simulink model "gnc_1__1_1"  (R2025b)
settings: Solver=VariableStepAuto  StartTime=0.0  StopTime=10.0  RelTol=1e-3
libraries: simulink_extras x4
settings Model: Creator=hp  LastModifiedBy=ADMIN

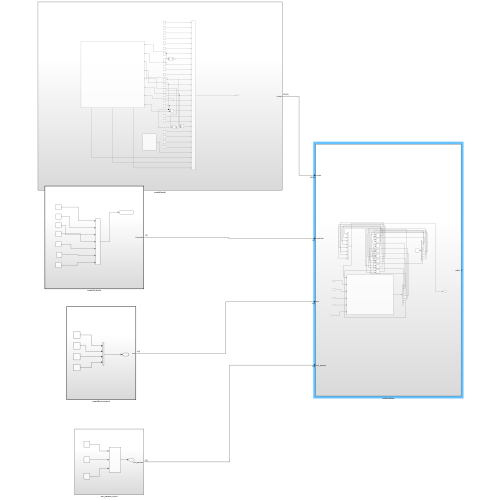
[thumbnail: Simulink's stored preview of the top-level diagram]
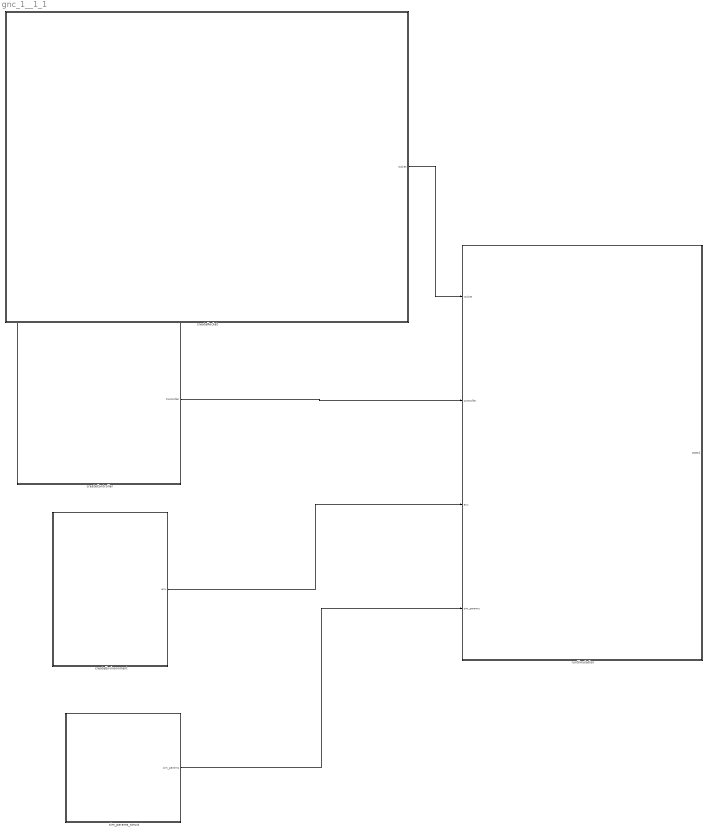
== system gnc_1__1_1 ==
  createController : Subsystem  TreatAsAtomicUnit=on
  createEnvironnment : Subsystem  TreatAsAtomicUnit=on
  createRocket : Subsystem
  runSimulation : Subsystem
  sim_params_struct : Subsystem
  wires:
  sim_params_struct/1(sim_params) -> runSimulation/4(sim_params)
  createEnvironnment/1(env) -> runSimulation/3(env)
  createController/1(Controller) -> runSimulation/2(controller)
  createRocket/1(rocket) -> runSimulation/1(rocket)

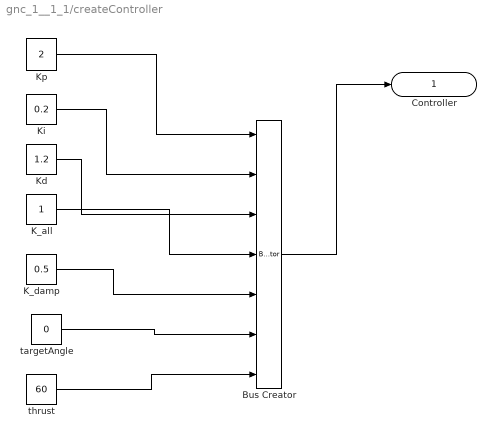
== system gnc_1__1_1/createController ==
  Bus Creator : BusCreator  Inputs=7
  K_all : Constant
  K_damp : Constant  Value=0.5
  Kd : Constant  Value=1.2
  Ki : Constant  Value=0.2
  Kp : Constant  Value=2
  targetAngle : Constant  Value=0
  thrust : Constant  Value=60
  Controller : Outport
  wires:
  Kp/1 -> Bus Creator/1
  Ki/1 -> Bus Creator/2
  Kd/1 -> Bus Creator/3
  K_all/1 -> Bus Creator/4
  K_damp/1 -> Bus Creator/5
  targetAngle/1 -> Bus Creator/6
  thrust/1 -> Bus Creator/7
  Bus Creator/1 -> Controller/1

== system gnc_1__1_1/createEnvironnment ==
  Bus Creator : BusCreator  Inputs=4
  P0 : Constant  Value=101325
  RHO0 : Constant  Value=1.225
  T0 : Constant  Value=288.15
  g : Constant  Value=9.81
  env : Outport
  wires:
  Bus Creator/1 -> env/1
  g/1 -> Bus Creator/1
  T0/1 -> Bus Creator/2
  P0/1 -> Bus Creator/3
  RHO0/1 -> Bus Creator/4

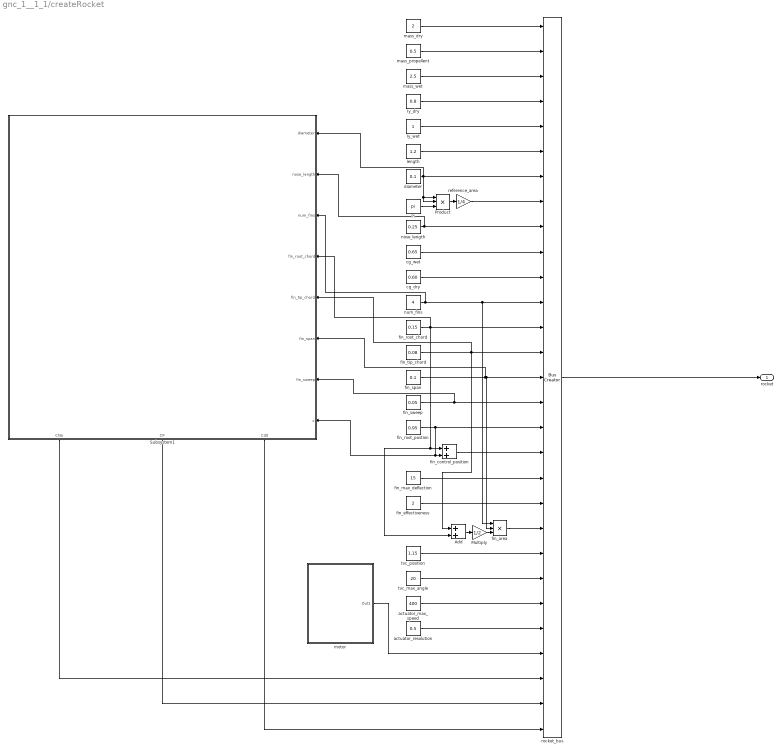
== system gnc_1__1_1/createRocket ==
  Add : Sum
  Iy_dry : Constant  Value=0.8
  Iy_wet : Constant
  Multiply : Gain  Gain=1/2
  Pi : Constant  Value=pi  OutDataTypeStr=Inherit: Inherit via back propagation
  Product : Product  Inputs=3
  Subsystem1 : Subsystem
      settings: PortSchema="{\"entries\":[{\"content\":{\"sides\":[{\"content\":{},\"type\":\"ConnectorPlacement.EquallySpacedRectSide\",\"uuid\":\"6679e0f2-b643-4e75-9411-8b79dd5cee92\"},{\"content\":{\"connectorIds\":[\"In1\",\"In2\",\"In3\",\"In4\",\"In5\",\"In6\",\"In7\",\"In8\"],\"side\":\"RIGHT\"},\"type\":\"ConnectorPlacement.EquallySpacedRectSide\",\"uuid\":\"6d3ac53c-a821-4766-a15e-70655263746a\"},{\"content\":{\"side\":\"TOP\"},\"type\":\"ConnectorPlacement.EquallySpacedRectSide\",\"uuid\":\"46e0cd8b-4eef-41f6-92b2-050981f5fcf1\"},{\"content\":{\"connectorIds\":[\"Out1\",\"Out2\",\"Out3\"],\"side\":\"BOTTOM\"},\"type\":\"ConnectorPlacement.EquallySpacedRectSide\",\"uuid\":\"5cd6cbdf-525c-430d-9c05-99018f0a78e6\"}]},\"type\":\"ConnectorPlacement.EquallySpacedConnector\",\"uuid\":\"94beb952-66d5-4b70-b8d3-e34f75b09e6c\"}],\"packageUris\":[\"http://schema.mathworks.com/mf0/Connector/R2020b\"],\"version\":\"1.0\"}"
  actuator_max_speed : Constant  Value=400
  actuator_resolution : Constant  Value=0.5
  cg_dry : Constant  Value=0.60
  cg_wet : Constant  Value=0.65
  diameter : Constant  Value=0.1
  fin_area : Product  Inputs=3
  fin_control_position : Sum
  fin_effectiveness : Constant  Value=2
  fin_max_deflection : Constant  Value=15
  fin_root_chord : Constant  Value=0.15
  fin_root_postion : Constant  Value=0.95
  fin_span : Constant  Value=0.1
  fin_sweep : Constant  Value=0.05
  fin_tip_chord : Constant  Value=0.08
  length : Constant  Value=1.2
  mass_dry : Constant  Value=2
  mass_propellent : Constant  Value=0.5
  mass_wet : Constant  Value=2.5
  motor : Subsystem
  nose_length : Constant  Value=0.25
  num_fins : Constant  Value=4
  reference_area : Gain  Gain=1/4
  rocket_bus : BusCreator  Inputs=29
  tvc_max_angle : Constant  Value=20
  tvc_position : Constant  Value=1.15
  rocket : Outport
  wires:
  Iy_wet/1 -> rocket_bus/5
  fin_tip_chord/1 -> Subsystem1/5(fin_tip_chord), rocket_bus/14, Add/1
  num_fins/1 -> Subsystem1/3(num_fins), fin_area/1, rocket_bus/12
  diameter/1 -> Subsystem1/1(diameter), rocket_bus/7, Product/1, Product/2
  fin_span/1 -> Subsystem1/6(fin_span), fin_area/2, rocket_bus/15
  mass_dry/1 -> rocket_bus/1
  Product/1 -> reference_area/1
  fin_sweep/1 -> Subsystem1/7(fin_sweep), rocket_bus/16
  fin_control_position/1 -> rocket_bus/18
  tvc_max_angle/1 -> rocket_bus/23
  rocket_bus/1 -> rocket/1
  Multiply/1 -> fin_area/3
  mass_propellent/1 -> rocket_bus/2
  fin_root_postion/1 -> Subsystem1/8(x), fin_control_position/2, rocket_bus/17
  fin_area/1 -> rocket_bus/21
  motor/1(Out1) -> rocket_bus/26
  Subsystem1/2(CP) -> rocket_bus/28
  Pi/1 -> Product/3
  tvc_position/1 -> rocket_bus/22
  cg_wet/1 -> rocket_bus/10
  fin_root_chord/1 -> Subsystem1/4(fin_root_chord), rocket_bus/13, fin_control_position/1, Add/2
  cg_dry/1 -> rocket_bus/11
  Iy_dry/1 -> rocket_bus/4
  actuator_max_speed/1 -> rocket_bus/24
  reference_area/1 -> rocket_bus/8
  Add/1 -> Multiply/1
  fin_max_deflection/1 -> rocket_bus/19
  length/1 -> rocket_bus/6
  fin_effectiveness/1 -> rocket_bus/20
  Subsystem1/3(Cd0) -> rocket_bus/29
  nose_length/1 -> Subsystem1/2(nose_length), rocket_bus/9
  mass_wet/1 -> rocket_bus/3
  actuator_resolution/1 -> rocket_bus/25
  Subsystem1/1(CNa) -> rocket_bus/27

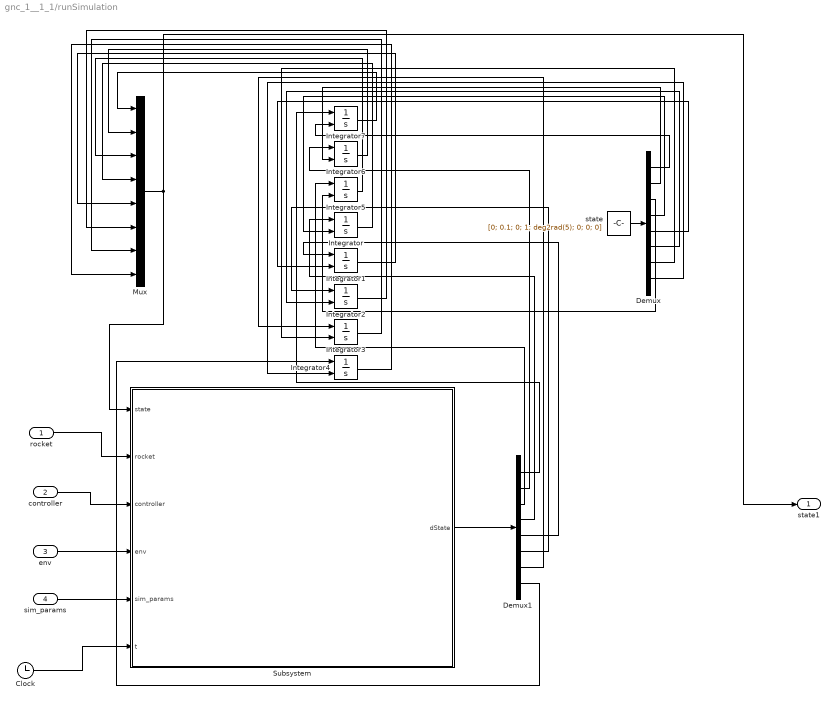
== system gnc_1__1_1/runSimulation ==
  rocket : Inport
  controller : Inport  Port=2
  env : Inport  Port=3
  sim_params : Inport  Port=4
  Clock : Clock
  Demux : Demux  Outputs=8
  Demux1 : Demux  Outputs=8
  Integrator : Integrator  InitialConditionSource=external  ContinuousStateAttributes=vz
  Integrator1 : Integrator  InitialConditionSource=external  ContinuousStateAttributes=theta
  Integrator2 : Integrator  InitialConditionSource=external  ContinuousStateAttributes=omega
  Integrator3 : Integrator  InitialConditionSource=external  ContinuousStateAttributes=actuator_angle
  Integrator4 : Integrator  InitialConditionSource=external  ContinuousStateAttributes=int_error
  Integrator5 : Integrator  InitialConditionSource=external  ContinuousStateAttributes=vx
  Integrator6 : Integrator  InitialConditionSource=external  ContinuousStateAttributes=z
  Integrator7 : Integrator  InitialConditionSource=external  ContinuousStateAttributes=x
  Mux : Mux  Inputs=8
  Subsystem : Subsystem
  state : Constant  Value=[0; 0.1; 0; 1; deg2rad(5); 0; 0; 0]
  state1 : Outport
  wires:
  rocket/1 -> Subsystem/2(rocket)
  controller/1 -> Subsystem/3(controller)
  env/1 -> Subsystem/4(env)
  sim_params/1 -> Subsystem/5(sim_params)
  Clock/1 -> Subsystem/6(t)
  Subsystem/1(dState) -> Demux1/1
  state/1 -> Demux/1
  Demux1/1 -> Integrator7/1
  Demux/1 -> Integrator7/2
  Demux1/2 -> Integrator6/1
  Demux/2 -> Integrator6/2
  Demux/3 -> Integrator5/2
  Demux1/3 -> Integrator5/1
  Demux/4 -> Integrator/2
  Demux1/4 -> Integrator/1
  Demux/5 -> Integrator1/2
  Demux1/5 -> Integrator1/1
  Demux/6 -> Integrator2/2
  Demux1/6 -> Integrator2/1
  Demux/7 -> Integrator3/2
  Demux1/7 -> Integrator3/1
  Demux/8 -> Integrator4/2
  Demux1/8 -> Integrator4/1
  Integrator7/1 -> Mux/1
  Integrator6/1 -> Mux/2
  Integrator5/1 -> Mux/3
  Integrator/1 -> Mux/4
  Integrator1/1 -> Mux/5
  Integrator2/1 -> Mux/6
  Integrator3/1 -> Mux/7
  Integrator4/1 -> Mux/8
  Mux/1 -> Subsystem/1(state), state1/1

== system gnc_1__1_1/sim_params_struct ==
  Bus Creator : BusCreator  Inputs=3
  dt : Constant  Value=0.0005
  launch_time : Constant  Value=0.5
  max_time : Constant  Value=45
  sim_params : Outport
  wires:
  dt/1 -> Bus Creator/1
  max_time/1 -> Bus Creator/2
  launch_time/1 -> Bus Creator/3
  Bus Creator/1 -> sim_params/1

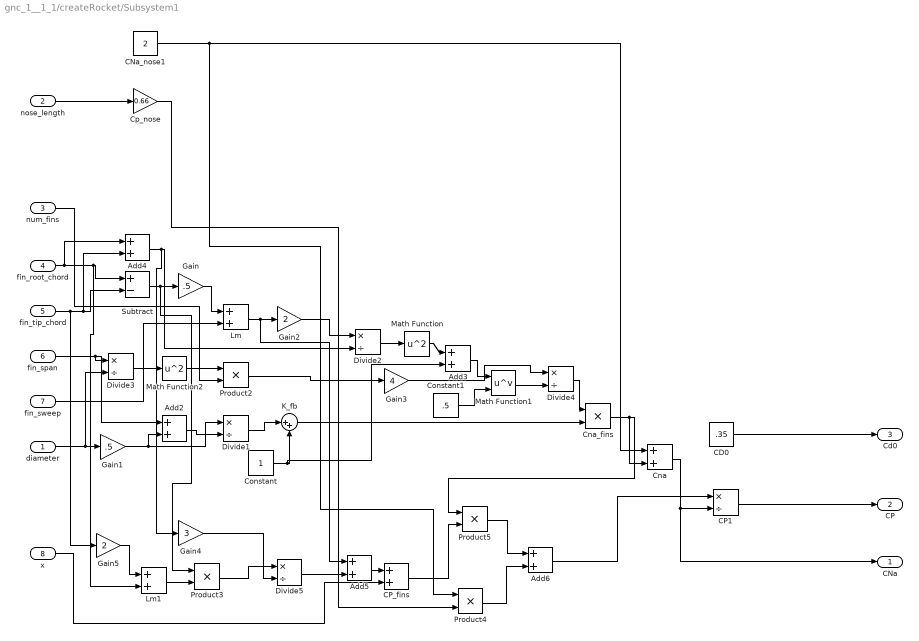
== system gnc_1__1_1/createRocket/Subsystem1 ==
  diameter : Inport
  nose_length : Inport  Port=2
  num_fins : Inport  Port=3
  fin_root_chord : Inport  Port=4
  fin_tip_chord : Inport  Port=5
  fin_span : Inport  Port=6
  fin_sweep : Inport  Port=7
  x : Inport  Port=8
  Add{2..6} (5 alike) : Sum
  CD0 : Constant  Value=.35
  CNa_nose1 : Constant  Value=2
  CP1 : Product  Inputs=*/
  CP_fins : Sum
  Cna : Sum
  Cna_fins : Product
  Constant : Constant
  Constant1 : Constant  Value=.5
  Cp_nose : Gain  Gain=0.66
  Divide{1..5} (5 alike) : Product  Inputs=*/
  Gain : Gain  Gain=.5
  Gain1 : Gain  Gain=.5
  Gain2 : Gain  Gain=2
  Gain3 : Gain  Gain=4
  Gain4 : Gain  Gain=3
  Gain5 : Gain  Gain=2
  K_fb : Sum  Inputs=|++
  Lm : Sum
  Lm1 : Sum
  Math Function : Math  Operator=square
  Math Function1 : Math  Operator=pow
  Math Function2 : Math  Operator=square
  Product{2..5} (4 alike) : Product
  Subtract : Sum  Inputs=+-
  CNa : Outport
  CP : Outport  Port=2
  Cd0 : Outport  Port=3
  wires:
  Cna/1 -> CNa/1, CP1/2
  Gain/1 -> Lm/1
  CP1/1 -> CP/1
  Gain2/1 -> Divide2/1
  nose_length/1 -> Cp_nose/1
  Divide2/1 -> Math Function/1
  Add5/1 -> CP_fins/1
  Math Function/1 -> Add3/1
  Constant1/1 -> Math Function1/2
  CNa_nose1/1 -> Product4/1, Cna/1
  CP_fins/1 -> Product5/2
  Divide1/1 -> K_fb/1
  Divide3/1 -> Math Function2/1
  Gain4/1 -> Divide5/2
  fin_span/1 -> Divide3/1, Add2/1
  Lm1/1 -> Product3/2
  Gain1/1 -> Divide1/1, Add2/2
  Divide5/1 -> Add5/2
  fin_sweep/1 -> Lm/2
  Add3/1 -> Math Function1/1
  Add6/1 -> CP1/1
  Gain5/1 -> Lm1/1
  Add4/1 -> Gain4/1, Divide2/2
  fin_root_chord/1 -> Add4/1, Lm1/2, Subtract/1
  CD0/1 -> Cd0/1
  Divide4/1 -> Cna_fins/1
  Subtract/1 -> Product3/1, Gain/1
  x/1 -> CP_fins/2
  Math Function2/1 -> Product2/1
  Product3/1 -> Divide5/1
  Product2/1 -> Gain3/1
  Product5/1 -> Add6/1
  Add2/1 -> Divide1/2
  Math Function1/1 -> Divide4/2
  Constant/1 -> Add3/2, K_fb/2
  Cp_nose/1 -> Product4/2
  num_fins/1 -> Product2/2
  fin_tip_chord/1 -> Add4/2, Subtract/2, Gain5/1
  Cna_fins/1 -> Product5/1, Cna/2
  Gain3/1 -> Divide4/1
  diameter/1 -> Divide3/2, Gain1/1
  Lm/1 -> Add5/1, Gain2/1
  Product4/1 -> Add6/2
  K_fb/1 -> Cna_fins/2

== system gnc_1__1_1/createRocket/motor ==
  burn_time : Constant  Value=20
  motor : BusCreator  Inputs=4
  propellant_mass : Constant
  thrust : Constant  Value=[50, 50, 50, 50, 50, 50, 50, 50, 0, 0]
  time : Constant  Value=[0, 0.5, 2, 5, 10, 15, 18, 19.5, 20, 20.5]
  Out1 : Outport
  wires:
  burn_time/1 -> motor/1
  time/1 -> motor/3
  propellant_mass/1 -> motor/2
  thrust/1 -> motor/4
  motor/1 -> Out1/1

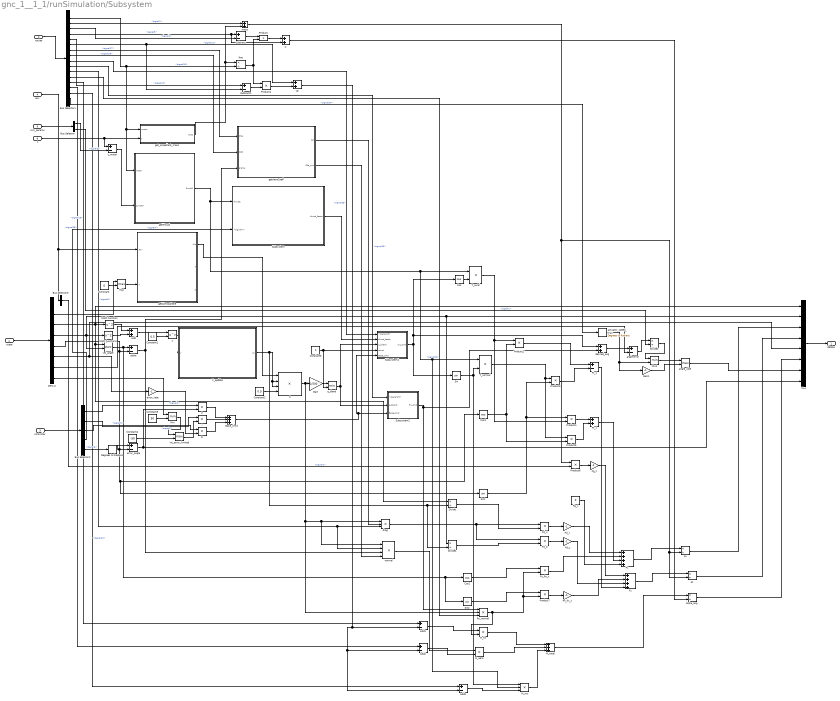
== system gnc_1__1_1/runSimulation/Subsystem ==
  state : Inport
  rocket : Inport  Port=2
  controller : Inport  Port=3
  env : Inport  Port=4
  sim_params : Inport  Port=5
  t : Inport  Port=6
  Add : Sum
  Add1 : Sum  Inputs=+-
  Add2 : Sum  Inputs=+-
  Add3 : Sum  Inputs=+-
  Base_Cmd : Sum  Inputs=+++
  Bus Selector : BusSelector  OutputSignals=signal3,signal1
  Bus Selector1 : BusSelector  OutputSignals=signal26,signal1,signal4,signal5,signal10,signal11,signal27,signal29,signal23,signal19,signal8,signal20,signal18,signal28,signal22,signal24
  Bus Selector2 : BusSelector  OutputSignals=signal1,signal2,signal3,signal7,signal6
  Bus Selector3 : BusSelector  OutputSignals=signal1
  Constant : Constant  Value=0
  Constant1 : Constant  Value=0.5
  Constant2 : Constant  Value=0.5
  Constant3 : Constant  Value=50
  Constant4 : Constant  Value=-50
  Constant5 : Constant
  Cos : Trigonometry  Operator=cos
  Cos1 : Trigonometry  Operator=cos
  Cos2 : Trigonometry  Operator=cos
  D : Product
  Degrees to Radians : simulink_extras/Transformations/Degrees to Radians
  Demux : Demux  Outputs=8
  Divide : Product  Inputs=*/
  Divide1 : Product  Inputs=*/
  Divide2 : Product  Inputs=*/
  Fd_X : Product
  Fd_Z : Product
  Fd_x : Gain  Gain=-1
  Fd_z : Gain  Gain=-1
  Fg_x : Constant  Value=0
  Fg_z : Gain  Gain=-1
  Fn_fin_x : Product
  Fn_fin_z : Gain  Gain=-1
  Ft_x : Sum
  Ft_z : Sum  Inputs=+-
  Fx : Sum  Inputs=++++
  Fz : Sum  Inputs=++++
  Gain : Gain  Gain=1/500
  Gain1 : Gain  Gain=-1
  I : Product
  Iy : Sum
  M_aero : Product
  M_fin : Product
  M_total : Sum  Inputs=+++
  M_tvc : Product  Inputs=3
  Math Function : Math  Operator=square
  Math Function1 : Math  Operator=square
  Max : MinMax  Function=max  Inputs=2
  Min : MinMax  Inputs=2
  Min1 : MinMax  Inputs=2
  Mux : Mux  Inputs=8
  P : Product
  Product{,1..7} (8 alike) : Product
  Sin : Trigonometry
  Sin1 : Trigonometry
  Sin2 : Trigonometry
  Subsystem : Subsystem
  Subsystem1 : Subsystem
  Subsystem2 : Subsystem
  Subtract : Sum  Inputs=+-
  Subtract1 : Sum  Inputs=+-
  T_axial : Product
  T_normal : Product
  V : Math  Operator=pow
  V_apdate : Subsystem
  actuator_speed_max : simulink_extras/Transformations/Degrees to Radians
  alpha : Sum  Inputs=+-
  alpha_ang : Product  Inputs=*/
  angle error : Sum  Inputs=+-
  angle_rate : MinMax  Function=max  Inputs=2
  ax : Product  Inputs=*/
  az : Product  Inputs=*/
  cg : Sum
  desired_ang : Sum
  drag : Product  Inputs=3
  error_angle : Sum  Inputs=+-
  error_rate : Gain  Gain=-1
  fin_normal : Product  Inputs=3
  frac : Product  Inputs=*/
  getAeroCoeff : Subsystem
  getAtmosphere : Subsystem
  getThrust : Subsystem
  get_propellant_mass : Subsystem
  int_error_limited : MinMax  Function=max  Inputs=2
  mass : Sum
  normal : Product  Inputs=4
  q : Product  Inputs=4
  q_blend : MinMax  Inputs=2
  t_motor : Sum  Inputs=+-
  vel_angle : Trigonometry  Operator=atan2
  dState : Outport
  wires:
  sim_params/1 -> Bus Selector/1
  rocket/1 -> Bus Selector1/1
  t/1 -> t_motor/1, get_propellant_mass/2(t)
  Bus Selector/1 -> t_motor/2  "<signal3>"
  Bus Selector1/1 -> getThrust/1(motor), get_propellant_mass/1(motor), frac/2  "<signal26>"
  get_propellant_mass/1(Out1) -> mass/2, frac/1
  Bus Selector1/2 -> mass/1  "<signal1>"
  Bus Selector1/4 -> Iy/2, Subtract/1  "<signal5>"
  Bus Selector1/3 -> Subtract/2  "<signal4>"
  frac/1 -> Product1/1, Product/2
  Subtract/1 -> Product/1
  Product/1 -> Iy/1
  Bus Selector1/5 -> Subtract1/1  "<signal10>"
  Bus Selector1/6 -> cg/1, Subtract1/2  "<signal11>"
  Subtract1/1 -> Product1/2
  Product1/1 -> cg/2
  t_motor/1 -> getThrust/2(t_motor)
  env/1 -> Bus Selector3/1, getAtmosphere/1(env)
  state/1 -> Demux/1
  Demux/2 -> Max/1
  Constant/1 -> Max/2
  Max/1 -> getAtmosphere/2(h)
  Demux/3 -> vel_angle/1, Divide/1, Math Function/1, Mux/1
  Demux/4 -> vel_angle/2, Math Function1/1, Divide1/1, Mux/2
  Math Function/1 -> Add/1
  Math Function1/1 -> Add/2
  Add/1 -> V/1
  Constant1/1 -> V/2
  V/1 -> V_apdate/1(V)
  vel_angle/1 -> Sin2/1, Cos2/1, alpha/1
  Demux/5 -> Sin1/1, Cos1/1, error_angle/2, alpha/2
  Bus Selector1/7 -> getAeroCoeff/1(CNa)  "<signal27>"
  Bus Selector1/8 -> getAeroCoeff/2(Cd0)  "<signal29>"
  alpha/1 -> normal/3, getAeroCoeff/3(alpha)
  V_apdate/1(V1) -> Divide1/2, Divide/2, q/3, q/2
  getAtmosphere/1(rho) -> q/1
  Constant2/1 -> q/4
  controller/1 -> Bus Selector2/1
  Bus Selector2/1 -> P/1  "<signal1>"
  Bus Selector2/2 -> I/1  "<signal2>"
  Bus Selector2/5 -> Degrees to Radians/1  "<signal6>"
  Degrees to Radians/1 -> error_angle/1
  Demux/8 -> Min/1
  Constant3/1 -> Min/2
  Constant4/1 -> int_error_limited/2
  Min/1 -> int_error_limited/1
  error_angle/1 -> Mux/8, P/2
  int_error_limited/1 -> I/2
  Bus Selector2/3 -> D/1  "<signal3>"
  error_rate/1 -> D/2
  P/1 -> Base_Cmd/1
  I/1 -> Base_Cmd/2
  D/1 -> Base_Cmd/3
  q/1 -> normal/1, drag/1, fin_normal/2, Gain/1
  Gain/1 -> q_blend/1
  Constant5/1 -> Subsystem1/4(const), q_blend/2
  getThrust/1(thrust1) -> T_axial/1, M_tvc/2, T_normal/1, Subsystem/1(thrust1)
  Bus Selector2/4 -> Subsystem/2(<signal7>)  "<signal7>"
  Bus Selector1/9 -> Subsystem1/1(<signal23>)  "<signal23>"
  Subsystem/1(thrust_factor) -> Subsystem1/2(thrust_factor)
  q_blend/1 -> Subsystem2/2(q_blend), Subsystem1/3(q_blend)
  Base_Cmd/1 -> Subsystem1/5(Base_cmd), Subsystem2/3(Base_cmd)
  Bus Selector1/10 -> Subsystem2/1(<signal19>)  "<signal19>"
  Subsystem1/1(tvc_cmd) -> desired_ang/1, Cos/1, Sin/1
  Cos/1 -> T_axial/2
  Sin/1 -> M_tvc/1, T_normal/2
  Cos1/1 -> Product2/2, Product5/2
  T_axial/1 -> Product2/1, Product4/2
  T_normal/1 -> Product5/1, Product3/1
  Product2/1 -> Ft_z/1
  Product3/1 -> Ft_z/2
  Sin1/1 -> Product4/1, Product3/2
  Product5/1 -> Ft_x/2
  Product4/1 -> Ft_x/1
  getAeroCoeff/1(Cd) -> drag/2
  Bus Selector1/11 -> normal/2, drag/3  "<signal8>"
  getAeroCoeff/2(CNa_out) -> normal/4
  drag/1 -> Fd_Z/1, Fd_X/1
  Divide/1 -> Fd_X/2
  Divide1/1 -> Fd_Z/2
  Fd_X/1 -> Fd_x/1
  Fd_Z/1 -> Fd_z/1
  Cos2/1 -> Fn_fin_x/1
  Sin2/1 -> Product7/1
  Product7/1 -> Fn_fin_z/1
  Bus Selector1/12 -> fin_normal/3  "<signal20>"
  Subsystem2/1(fin_cmd) -> fin_normal/1, desired_ang/2
  Bus Selector1/13 -> Add1/1  "<signal18>"
  cg/1 -> Add1/2, Add2/2, Add3/2
  Add1/1 -> M_fin/1
  Bus Selector1/14 -> Add2/1  "<signal28>"
  normal/1 -> M_aero/1
  Add2/1 -> M_aero/2
  Bus Selector1/15 -> Add3/1  "<signal22>"
  Add3/1 -> M_tvc/3
  M_fin/1 -> M_total/1
  M_aero/1 -> M_total/2
  M_tvc/1 -> M_total/3
  Fd_x/1 -> Fx/1
  Fn_fin_x/1 -> Fx/2
  Ft_x/1 -> Fx/3
  Fg_x/1 -> Fx/4
  mass/1 -> az/2, ax/2, Product6/1
  Bus Selector3/1 -> Product6/2  "<signal1>"
  Product6/1 -> Fg_z/1
  Fg_z/1 -> Fz/1
  Fn_fin_z/1 -> Fz/2
  Fd_z/1 -> Fz/3
  Ft_z/1 -> Fz/4
  Fx/1 -> ax/1
  Fz/1 -> az/1
  M_total/1 -> alpha_ang/1
  Iy/1 -> alpha_ang/2
  ax/1 -> Mux/3
  az/1 -> Mux/4
  Demux/6 -> Mux/5, error_rate/1
  alpha_ang/1 -> Mux/6
  angle_rate/1 -> Mux/7
  Bus Selector1/16 -> actuator_speed_max/1  "<signal24>"
  Demux/7 -> angle error/2
  desired_ang/1 -> angle error/1
  Bus Selector/2 -> Divide2/2  "<signal1>"
  angle error/1 -> Divide2/1
  Divide2/1 -> Min1/1
  actuator_speed_max/1 -> Gain1/1, Min1/2
  Gain1/1 -> angle_rate/2
  Min1/1 -> angle_rate/1
  Mux/1 -> dState/1
  fin_normal/1 -> M_fin/2, Fn_fin_x/2, Product7/2

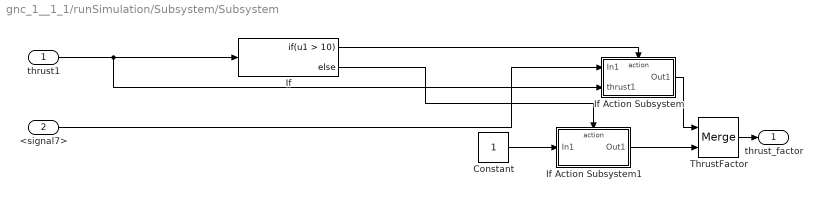
== system gnc_1__1_1/runSimulation/Subsystem/Subsystem ==
  thrust1 : Inport
  <signal7> : Inport  Port=2
  Constant : Constant
  If : If  IfExpression=u1 > 10
  If Action Subsystem : Subsystem  TreatAsAtomicUnit=on
  If Action Subsystem1 : Subsystem  TreatAsAtomicUnit=on
  ThrustFactor : Merge
  thrust_factor : Outport
  wires:
  If/1 -> If Action Subsystem/Action
  ThrustFactor/1 -> thrust_factor/1
  thrust1/1 -> If Action Subsystem/2(thrust1), If/1
  If/2 -> If Action Subsystem1/Action
  If Action Subsystem1/1(Out1) -> ThrustFactor/2
  <signal7>/1 -> If Action Subsystem/1(In1)
  If Action Subsystem/1(Out1) -> ThrustFactor/1
  Constant/1 -> If Action Subsystem1/1(In1)

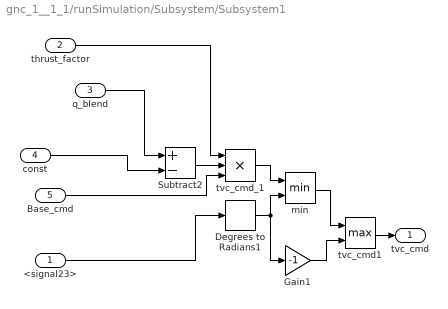
== system gnc_1__1_1/runSimulation/Subsystem/Subsystem1 ==
  <signal23> : Inport
  thrust_factor : Inport  Port=2
  q_blend : Inport  Port=3
  const : Inport  Port=4
  Base_cmd : Inport  Port=5
  Degrees to Radians1 : simulink_extras/Transformations/Degrees to Radians
  Gain1 : Gain  Gain=-1
  Subtract2 : Sum  Inputs=+-
  min : MinMax  Inputs=2
  tvc_cmd1 : MinMax  Function=max  Inputs=2
  tvc_cmd_1 : Product  Inputs=3
  tvc_cmd : Outport
  wires:
  Subtract2/1 -> tvc_cmd_1/2
  tvc_cmd_1/1 -> min/1
  tvc_cmd1/1 -> tvc_cmd/1
  Gain1/1 -> tvc_cmd1/2
  Base_cmd/1 -> tvc_cmd_1/3
  Degrees to Radians1/1 -> Gain1/1, min/2
  min/1 -> tvc_cmd1/1
  thrust_factor/1 -> tvc_cmd_1/1
  <signal23>/1 -> Degrees to Radians1/1
  const/1 -> Subtract2/2
  q_blend/1 -> Subtract2/1

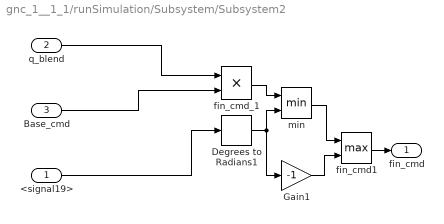
== system gnc_1__1_1/runSimulation/Subsystem/Subsystem2 ==
  <signal19> : Inport
  q_blend : Inport  Port=2
  Base_cmd : Inport  Port=3
  Degrees to Radians1 : simulink_extras/Transformations/Degrees to Radians
  Gain1 : Gain  Gain=-1
  fin_cmd1 : MinMax  Function=max  Inputs=2
  fin_cmd_1 : Product
  min : MinMax  Inputs=2
  fin_cmd : Outport
  wires:
  q_blend/1 -> fin_cmd_1/1
  <signal19>/1 -> Degrees to Radians1/1
  min/1 -> fin_cmd1/1
  Degrees to Radians1/1 -> Gain1/1, min/2
  Gain1/1 -> fin_cmd1/2
  fin_cmd1/1 -> fin_cmd/1
  fin_cmd_1/1 -> min/1
  Base_cmd/1 -> fin_cmd_1/2

== system gnc_1__1_1/runSimulation/Subsystem/V_apdate ==
  V : Inport
  If : If  IfExpression=u1 < 0.1
  If Action Subsystem : Subsystem  TreatAsAtomicUnit=on
  If Action Subsystem1 : Subsystem  TreatAsAtomicUnit=on
  Merge : Merge
  V1 : Outport
  wires:
  Merge/1 -> V1/1
  If/2 -> If Action Subsystem1/Action
  If Action Subsystem1/1(Out1) -> Merge/2
  If Action Subsystem/1(Out1) -> Merge/1
  V/1 -> If Action Subsystem1/1(In1), If/1
  If/1 -> If Action Subsystem/Action

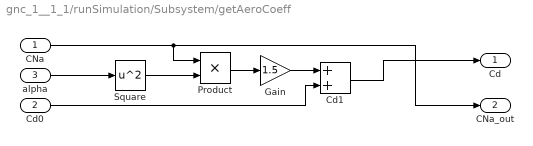
== system gnc_1__1_1/runSimulation/Subsystem/getAeroCoeff ==
  CNa : Inport
  Cd0 : Inport  Port=2
  alpha : Inport  Port=3
  Cd1 : Sum
  Gain : Gain  Gain=1.5
  Product : Product
  Square : Math  Operator=square
  Cd : Outport
  CNa_out : Outport  Port=2
  wires:
  alpha/1 -> Square/1
  CNa/1 -> CNa_out/1, Product/1
  Square/1 -> Product/2
  Product/1 -> Gain/1
  Gain/1 -> Cd1/1
  Cd0/1 -> Cd1/2
  Cd1/1 -> Cd/1

== system gnc_1__1_1/runSimulation/Subsystem/getAtmosphere ==
  env : Inport
  h : Inport  Port=2
  Bus Selector : BusSelector  OutputSignals=signal2,signal3
  MATLAB Function : MATLAB Function  TreatAsAtomicUnit=on
  rho : Outport
  T : Outport  Port=2
  P : Outport  Port=3
  wires:
  env/1 -> Bus Selector/1
  Bus Selector/1 -> MATLAB Function/1(T0)  "<signal2>"
  Bus Selector/2 -> MATLAB Function/2(P0)  "<signal3>"
  h/1 -> MATLAB Function/3(h)
  MATLAB Function/1(rho) -> rho/1
  MATLAB Function/2(T) -> T/1
  MATLAB Function/3(P) -> P/1

== system gnc_1__1_1/runSimulation/Subsystem/getThrust ==
  motor : Inport
  t_motor : Inport  Port=2
  Bus Selector : BusSelector  OutputSignals=signal3,signal4
  MATLAB Function : MATLAB Function  TreatAsAtomicUnit=on
  thrust1 : Outport
  wires:
  motor/1 -> Bus Selector/1
  t_motor/1 -> MATLAB Function/3(t)
  Bus Selector/1 -> MATLAB Function/1(time)  "<signal3>"
  Bus Selector/2 -> MATLAB Function/2(thrust)  "<signal4>"
  MATLAB Function/1(thrust1) -> thrust1/1

== system gnc_1__1_1/runSimulation/Subsystem/get_propellant_mass ==
  motor : Inport
  t : Inport  Port=2
  Bus Selector : BusSelector  OutputSignals=signal1,signal2
  Subsystem : Subsystem
  Out1 : Outport
  wires:
  motor/1 -> Bus Selector/1
  Bus Selector/1 -> Subsystem/2(burn_time)  "<signal1>"
  Bus Selector/2 -> Subsystem/3(propellant_mass)  "<signal2>"
  t/1 -> Subsystem/1(t)
  Subsystem/1(Out1) -> Out1/1

== system gnc_1__1_1/runSimulation/Subsystem/Subsystem/If Action Subsystem ==
  In1 : Inport
  thrust1 : Inport  Port=2
  Action Port : ActionPort  ActionPortLabel=if(u1 > 10)
  Divide : Product  Inputs=*/
  Out1 : Outport
  wires:
  In1/1 -> Divide/1
  thrust1/1 -> Divide/2
  Divide/1 -> Out1/1

== system gnc_1__1_1/runSimulation/Subsystem/Subsystem/If Action Subsystem1 ==
  In1 : Inport
  Action Port : ActionPort  ActionPortLabel=else
  Out1 : Outport
  wires:
  In1/1 -> Out1/1

== system gnc_1__1_1/runSimulation/Subsystem/V_apdate/If Action Subsystem ==
  Action Port : ActionPort  ActionPortLabel=if(u1 < 0.1)
  Constant : Constant  Value=0.1
  Out1 : Outport
  wires:
  Constant/1 -> Out1/1

== system gnc_1__1_1/runSimulation/Subsystem/V_apdate/If Action Subsystem1 ==
  In1 : Inport
  Action Port : ActionPort  ActionPortLabel=else
  Out1 : Outport
  wires:
  In1/1 -> Out1/1

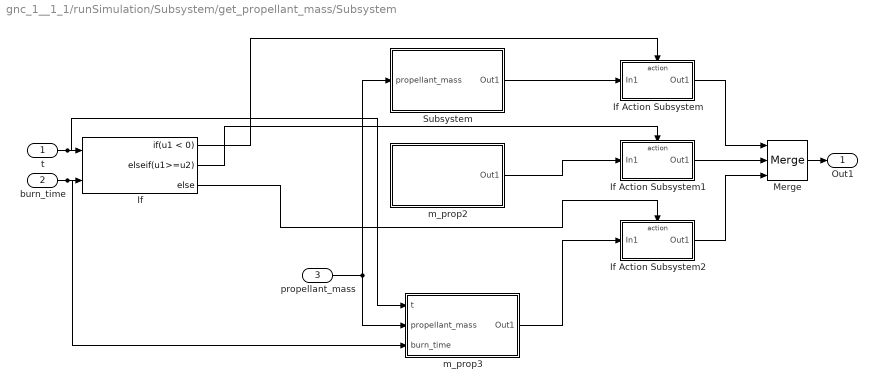
== system gnc_1__1_1/runSimulation/Subsystem/get_propellant_mass/Subsystem ==
  t : Inport
  burn_time : Inport  Port=2
  propellant_mass : Inport  Port=3
  If : If  NumInputs=2  IfExpression=u1 < 0  ElseIfExpressions=u1>=u2
  If Action Subsystem : Subsystem  TreatAsAtomicUnit=on
  If Action Subsystem1 : Subsystem  TreatAsAtomicUnit=on
  If Action Subsystem2 : Subsystem  TreatAsAtomicUnit=on
  Merge : Merge  Inputs=3
  Subsystem : Subsystem
  m_prop2 : Subsystem
  m_prop3 : Subsystem
  Out1 : Outport
  wires:
  propellant_mass/1 -> Subsystem/1(propellant_mass), m_prop3/2(propellant_mass)
  t/1 -> m_prop3/1(t), If/1
  If/3 -> If Action Subsystem2/Action
  If/1 -> If Action Subsystem/Action
  Subsystem/1(Out1) -> If Action Subsystem/1(In1)
  m_prop2/1(Out1) -> If Action Subsystem1/1(In1)
  If/2 -> If Action Subsystem1/Action
  burn_time/1 -> m_prop3/3(burn_time), If/2
  m_prop3/1(Out1) -> If Action Subsystem2/1(In1)
  If Action Subsystem/1(Out1) -> Merge/1
  If Action Subsystem1/1(Out1) -> Merge/2
  If Action Subsystem2/1(Out1) -> Merge/3
  Merge/1 -> Out1/1

== system gnc_1__1_1/runSimulation/Subsystem/get_propellant_mass/Subsystem/If Action Subsystem ==
  In1 : Inport
  Action Port : ActionPort  ActionPortLabel=if(u1 < 0)
  Out1 : Outport
  wires:
  In1/1 -> Out1/1

== system gnc_1__1_1/runSimulation/Subsystem/get_propellant_mass/Subsystem/If Action Subsystem1 ==
  In1 : Inport
  Action Port : ActionPort  ActionPortLabel=elseif(u1>=u2)
  Out1 : Outport
  wires:
  In1/1 -> Out1/1

== system gnc_1__1_1/runSimulation/Subsystem/get_propellant_mass/Subsystem/If Action Subsystem2 ==
  In1 : Inport
  Action Port : ActionPort  ActionPortLabel=else
  Out1 : Outport
  wires:
  In1/1 -> Out1/1

== system gnc_1__1_1/runSimulation/Subsystem/get_propellant_mass/Subsystem/Subsystem ==
  propellant_mass : Inport
  Out1 : Outport
  wires:
  propellant_mass/1 -> Out1/1

== system gnc_1__1_1/runSimulation/Subsystem/get_propellant_mass/Subsystem/m_prop2 ==
  Constant : Constant  Value=0
  Out1 : Outport
  wires:
  Constant/1 -> Out1/1

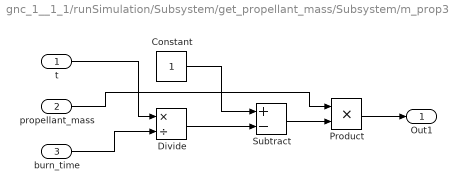
== system gnc_1__1_1/runSimulation/Subsystem/get_propellant_mass/Subsystem/m_prop3 ==
  t : Inport
  propellant_mass : Inport  Port=2
  burn_time : Inport  Port=3
  Constant : Constant
  Divide : Product  Inputs=*/
  Product : Product
  Subtract : Sum  Inputs=+-
  Out1 : Outport
  wires:
  t/1 -> Divide/1
  burn_time/1 -> Divide/2
  Constant/1 -> Subtract/1
  Divide/1 -> Subtract/2
  Subtract/1 -> Product/2
  propellant_mass/1 -> Product/1
  Product/1 -> Out1/1

== matlab function gnc_1__1_1/runSimulation/Subsystem/getAtmosphere/MATLAB Function ==
  data: T0 input; rho output; P0 input; h input; T output; P output
function [rho, T, P] = getAtmosphere(T0,P0, h)
    T = T0 - 0.0065 * h;
    if T < 216.65
        T = 216.65;
    end
    P = P0 * (T / T0)^5.255;
    rho = P / (287.05 * T);
end

== matlab function gnc_1__1_1/runSimulation/Subsystem/getThrust/MATLAB Function ==
  data: time input; thrust input; thrust1 output; t input
function thrust1 = getThrust(time, thrust, t)
    if t < 0 || t > time(end)
        thrust1 = 0;
    else
        thrust1 = interp1(time, thrust, t, 'linear');
    end
end
